simulink model "provaODE45_Simulink"  (R2020b)
settings: Solver=VariableStepAuto  StartTime=0.0  StopTime=30  MaxStep=0.01  RelTol=1e-3
values from neighbouring files (symbols this model uses):
  b = []    [I_GA.m]    (also in SIR_GA.m; autoSEIR_GA.m; autoSIR_GA.m; autofitness_fun.m = x(2))
  f = 1.8    [provaODE45.m]
  N = 60e6    (= 60000000)    [SIR_GA.m]    (also in autoSEIR_GA.m = 59999771; autoSIR_GA.m = 59999771; provaODE45.m = 10000; simulationSEIR.m = 600000)
  y0 = [Jv(length(J),1),Jv(length(J),2),Jv(length(J),3)]    [SIR_GA.m]    (also in autoSEIR_GA.m = [Jv(length(J),1),Jv(length(J),2),Jv(length(J),3),Jv(length(J; autoSIR_GA.m; fitness_fun.m = [N 1 0]; provaODE45.m = [N 1 0])
settings Model: Creator=abd99  LastModifiedBy=abd99

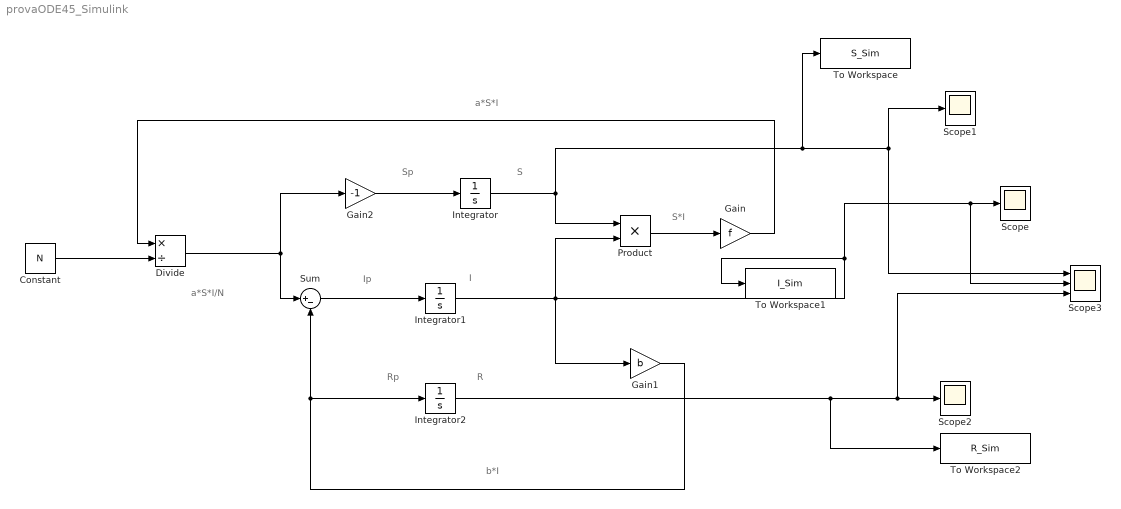
== system provaODE45_Simulink ==
  note: Ip
  note: I
  note: Sp
  note: S
  note: Rp
  note: R
  note: S*I
  note: a*S*I
  note: b*I
  note: a*S*I/N
  Constant : Constant  Value=N
  Divide : Product  Inputs=*/
  Gain : Gain  Gain=f
  Gain1 : Gain  Gain=b
  Gain2 : Gain  Gain=-1
  Integrator : Integrator  InitialCondition=N  UpperSaturationLimit=N  LowerSaturationLimit=0
  Integrator1 : Integrator  InitialCondition=y0(2)
  Integrator2 : Integrator  UpperSaturationLimit=N  LowerSaturationLimit=0
  Product : Product
  Scope : Scope
  Scope1 : Scope
  Scope2 : Scope
  Scope3 : Scope  NumInputPorts=3
  Sum : Sum  Inputs=|+-
  To Workspace : ToWorkspace  VariableName=S_Sim  SampleTime=-1
  To Workspace1 : ToWorkspace  VariableName=I_Sim  SampleTime=-1
  To Workspace2 : ToWorkspace  VariableName=R_Sim  SampleTime=-1
  wires:
  Integrator/1 -> To Workspace/1, Scope3/1, Scope1/1, Product/1
  Integrator1/1 -> Product/2, Scope3/2, Scope/1, To Workspace1/1, Gain1/1
  Product/1 -> Gain/1
  Sum/1 -> Integrator1/1
  Constant/1 -> Divide/2
  Integrator2/1 -> To Workspace2/1, Scope3/3, Scope2/1
  Gain1/1 -> Integrator2/1, Sum/2
  Divide/1 -> Gain2/1, Sum/1
  Gain/1 -> Divide/1
  Gain2/1 -> Integrator/1
